simulink model "Ground_Control_SC"  (R2020b)
settings: Solver=VariableStepAuto  StartTime=0.0  StopTime=10.0  RelTol=1e-3
settings Model: Creator=macra  LastModifiedBy=macra

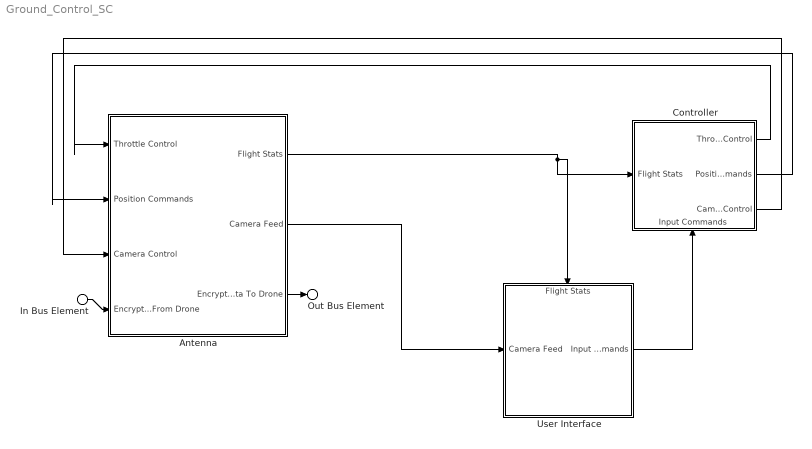
== system Ground_Control_SC ==
  In Bus Element : Inport  PortName=Encrypted Data From Drone
  Antenna : Subsystem
      settings: PortSchema="{\"entries\":[{\"content\":{\"headerSize\":26,\"margin\":15,\"minimumSpacing\":25,\"sides\":[{\"content\":{\"connectorIds\":[\"In1\",\"In2\",\"In3\",\"In4\"]},\"type\":\"ConnectorPlacement.EquallySpacedRectSide\",\"uuid\":\"8f51257f-f627-4f58-a4af-3e0fb88ba4bc\"},{\"content\":{\"connectorIds\":[\"Out1\",\"Out2\",\"Out3\"],\"side\":\"RIGHT\"},\"type\":\"ConnectorPlacement.EquallySpacedRectSide\",\"uuid\":\"f1fa1950-8e47-40b7-8d13-b3d0804be378\"},{\"content\":{\"connectorIds\":[],\"side\":\"TOP\"},\"type\":\"ConnectorPlacement.EquallySpacedRectSide\",\"uuid\":\"7a27bdc2-dc0c-4d7e-ba2c-0c757f448581\"},{\"content\":{\"connectorIds\":[],\"side\":\"HIDDEN\"},\"type\":\"ConnectorPlacement.EquallySpacedRectSide\",\"uuid\":\"bf1e85f7-7c79-4931-85e3-188682710bd5\"}]},\"type\":\"ConnectorPlacement.EquallySpacedConnector\",\"uuid\":\"5f8c8835-300e-4f03-b548-6a322d546785\"}],\"packageUris\":[\"http://schema.mathworks.com/mf0/Connector/R2020b\"],\"version\":\"1.0\"}"
  Controller : Subsystem
      settings: PortSchema="{\"entries\":[{\"content\":{\"headerSize\":26,\"margin\":15,\"minimumSpacing\":25,\"sides\":[{\"content\":{\"connectorIds\":[\"In1\"]},\"type\":\"ConnectorPlacement.EquallySpacedRectSide\",\"uuid\":\"8f51257f-f627-4f58-a4af-3e0fb88ba4bc\"},{\"content\":{\"connectorIds\":[\"Out1\",\"Out2\",\"Out3\"],\"side\":\"RIGHT\"},\"type\":\"ConnectorPlacement.EquallySpacedRectSide\",\"uuid\":\"f1fa1950-8e47-40b7-8d13-b3d0804be378\"},{\"content\":{\"connectorIds\":[],\"side\":\"TOP\"},\"type\":\"ConnectorPlacement.EquallySpacedRectSide\",\"uuid\":\"7a27bdc2-dc0c-4d7e-ba2c-0c757f448581\"},{\"content\":{\"connectorIds\":[\"In2\"],\"side\":\"BOTTOM\"},\"type\":\"ConnectorPlacement.EquallySpacedRectSide\",\"uuid\":\"100c20a7-19a0-4abc-9a19-4a6d998db79c\"},{\"content\":{\"connectorIds\":[],\"side\":\"HIDDEN\"},\"type\":\"ConnectorPlacement.EquallySpacedRectSide\",\"uuid\":\"bf1e85f7-7c79-4931-85e3-188682710bd5\"}]},\"type\":\"ConnectorPlacement.EquallySpacedConnector\",\"uuid\":\"5f8c8835-300e-4f03-b548-6a322d546785\"}],\"packageUris\":[\"http://schema.mathworks.com/mf0/Connector/R2020b\"],\"version\":\"1.0\"}"
  User Interface : Subsystem
      settings: PortSchema="{\"entries\":[{\"content\":{\"headerSize\":26,\"margin\":15,\"minimumSpacing\":25,\"sides\":[{\"content\":{\"connectorIds\":[\"In2\"]},\"type\":\"ConnectorPlacement.EquallySpacedRectSide\",\"uuid\":\"8f51257f-f627-4f58-a4af-3e0fb88ba4bc\"},{\"content\":{\"connectorIds\":[\"Out1\"],\"side\":\"RIGHT\"},\"type\":\"ConnectorPlacement.EquallySpacedRectSide\",\"uuid\":\"f1fa1950-8e47-40b7-8d13-b3d0804be378\"},{\"content\":{\"connectorIds\":[\"In1\"],\"side\":\"TOP\"},\"type\":\"ConnectorPlacement.EquallySpacedRectSide\",\"uuid\":\"7a27bdc2-dc0c-4d7e-ba2c-0c757f448581\"},{\"content\":{\"connectorIds\":[],\"side\":\"HIDDEN\"},\"type\":\"ConnectorPlacement.EquallySpacedRectSide\",\"uuid\":\"bf1e85f7-7c79-4931-85e3-188682710bd5\"}]},\"type\":\"ConnectorPlacement.EquallySpacedConnector\",\"uuid\":\"5f8c8835-300e-4f03-b548-6a322d546785\"}],\"packageUris\":[\"http://schema.mathworks.com/mf0/Connector/R2020b\"],\"version\":\"1.0\"}"
  Out Bus Element : Outport  PortName=Encrypted Data To Drone
  wires:
  Antenna/2(Camera Feed) -> User Interface/2(Camera Feed)
  User Interface/1(Input Commands) -> Controller/2(Input Commands)
  In Bus Element/1 -> Antenna/4(Encrypted Data From Drone)
  Antenna/3(Encrypted Data To Drone) -> Out Bus Element/1
  Antenna/1(Flight Stats) -> Controller/1(Flight Stats), User Interface/1(Flight Stats)
  Controller/1(Throttle Control) -> Antenna/1(Throttle Control)
  Controller/3(Camera Control) -> Antenna/3(Camera Control)
  Controller/2(Position Commands) -> Antenna/2(Position Commands)

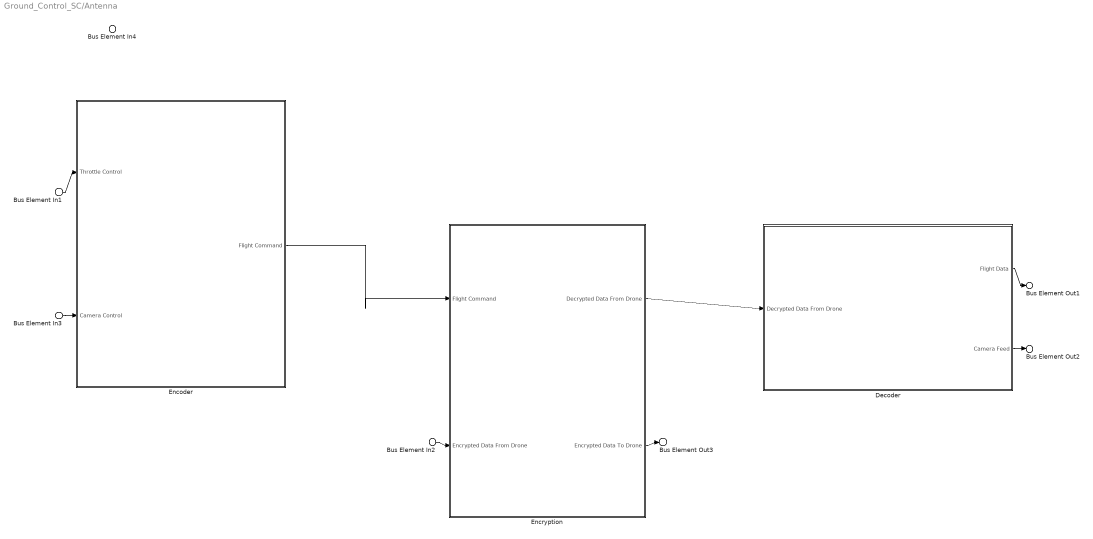
== system Ground_Control_SC/Antenna ==
  Bus Element In1 : Inport  PortName=Throttle Control
  Bus Element In4 : Inport  Port=2  PortName=Position Commands
  Bus Element In3 : Inport  Port=3  PortName=Camera Control
  Bus Element In2 : Inport  Port=4  PortName=Encrypted Data From Drone
  Decoder : Subsystem
      settings: PortSchema="{\"entries\":[{\"content\":{\"headerSize\":26,\"margin\":15,\"minimumSpacing\":25,\"sides\":[{\"content\":{\"connectorIds\":[\"In1\"]},\"type\":\"ConnectorPlacement.EquallySpacedRectSide\",\"uuid\":\"8f51257f-f627-4f58-a4af-3e0fb88ba4bc\"},{\"content\":{\"connectorIds\":[\"Out1\",\"Out2\"],\"side\":\"RIGHT\"},\"type\":\"ConnectorPlacement.EquallySpacedRectSide\",\"uuid\":\"f1fa1950-8e47-40b7-8d13-b3d0804be378\"},{\"content\":{\"connectorIds\":[],\"side\":\"TOP\"},\"type\":\"ConnectorPlacement.EquallySpacedRectSide\",\"uuid\":\"7a27bdc2-dc0c-4d7e-ba2c-0c757f448581\"},{\"content\":{\"connectorIds\":[],\"side\":\"HIDDEN\"},\"type\":\"ConnectorPlacement.EquallySpacedRectSide\",\"uuid\":\"bf1e85f7-7c79-4931-85e3-188682710bd5\"}]},\"type\":\"ConnectorPlacement.EquallySpacedConnector\",\"uuid\":\"5f8c8835-300e-4f03-b548-6a322d546785\"}],\"packageUris\":[\"http://schema.mathworks.com/mf0/Connector/R2020b\"],\"version\":\"1.0\"}"
  Encoder : Subsystem
      settings: PortSchema="{\"entries\":[{\"content\":{\"headerSize\":26,\"margin\":15,\"minimumSpacing\":25,\"sides\":[{\"content\":{\"connectorIds\":[\"In1\",\"In2\"]},\"type\":\"ConnectorPlacement.EquallySpacedRectSide\",\"uuid\":\"8f51257f-f627-4f58-a4af-3e0fb88ba4bc\"},{\"content\":{\"connectorIds\":[\"Out1\"],\"side\":\"RIGHT\"},\"type\":\"ConnectorPlacement.EquallySpacedRectSide\",\"uuid\":\"f1fa1950-8e47-40b7-8d13-b3d0804be378\"},{\"content\":{\"connectorIds\":[],\"side\":\"TOP\"},\"type\":\"ConnectorPlacement.EquallySpacedRectSide\",\"uuid\":\"7a27bdc2-dc0c-4d7e-ba2c-0c757f448581\"},{\"content\":{\"connectorIds\":[],\"side\":\"HIDDEN\"},\"type\":\"ConnectorPlacement.EquallySpacedRectSide\",\"uuid\":\"bf1e85f7-7c79-4931-85e3-188682710bd5\"}]},\"type\":\"ConnectorPlacement.EquallySpacedConnector\",\"uuid\":\"5f8c8835-300e-4f03-b548-6a322d546785\"}],\"packageUris\":[\"http://schema.mathworks.com/mf0/Connector/R2020b\"],\"version\":\"1.0\"}"
  Encryption : Subsystem
      settings: PortSchema="{\"entries\":[{\"content\":{\"headerSize\":26,\"margin\":15,\"minimumSpacing\":25,\"sides\":[{\"content\":{\"connectorIds\":[\"In1\",\"In2\"]},\"type\":\"ConnectorPlacement.EquallySpacedRectSide\",\"uuid\":\"8f51257f-f627-4f58-a4af-3e0fb88ba4bc\"},{\"content\":{\"connectorIds\":[\"Out1\",\"Out2\"],\"side\":\"RIGHT\"},\"type\":\"ConnectorPlacement.EquallySpacedRectSide\",\"uuid\":\"f1fa1950-8e47-40b7-8d13-b3d0804be378\"},{\"content\":{\"connectorIds\":[],\"side\":\"TOP\"},\"type\":\"ConnectorPlacement.EquallySpacedRectSide\",\"uuid\":\"7a27bdc2-dc0c-4d7e-ba2c-0c757f448581\"},{\"content\":{\"connectorIds\":[],\"side\":\"HIDDEN\"},\"type\":\"ConnectorPlacement.EquallySpacedRectSide\",\"uuid\":\"bf1e85f7-7c79-4931-85e3-188682710bd5\"}]},\"type\":\"ConnectorPlacement.EquallySpacedConnector\",\"uuid\":\"5f8c8835-300e-4f03-b548-6a322d546785\"}],\"packageUris\":[\"http://schema.mathworks.com/mf0/Connector/R2020b\"],\"version\":\"1.0\"}"
  Bus Element Out1 : Outport  PortName=Flight Stats
  Bus Element Out2 : Outport  Port=2  PortName=Camera Feed
  Bus Element Out3 : Outport  Port=3  PortName=Encrypted Data To Drone
  wires:
  Bus Element In2/1 -> Encryption/2(Encrypted Data From Drone)
  Encryption/2(Encrypted Data To Drone) -> Bus Element Out3/1
  Encryption/1(Decrypted Data From Drone) -> Decoder/1(Decrypted Data From Drone)
  Decoder/1(Flight Data) -> Bus Element Out1/1
  Decoder/2(Camera Feed) -> Bus Element Out2/1
  Encoder/1(Flight Command) -> Encryption/1(Flight Command)
  Bus Element In1/1 -> Encoder/1(Throttle Control)
  Bus Element In3/1 -> Encoder/2(Camera Control)

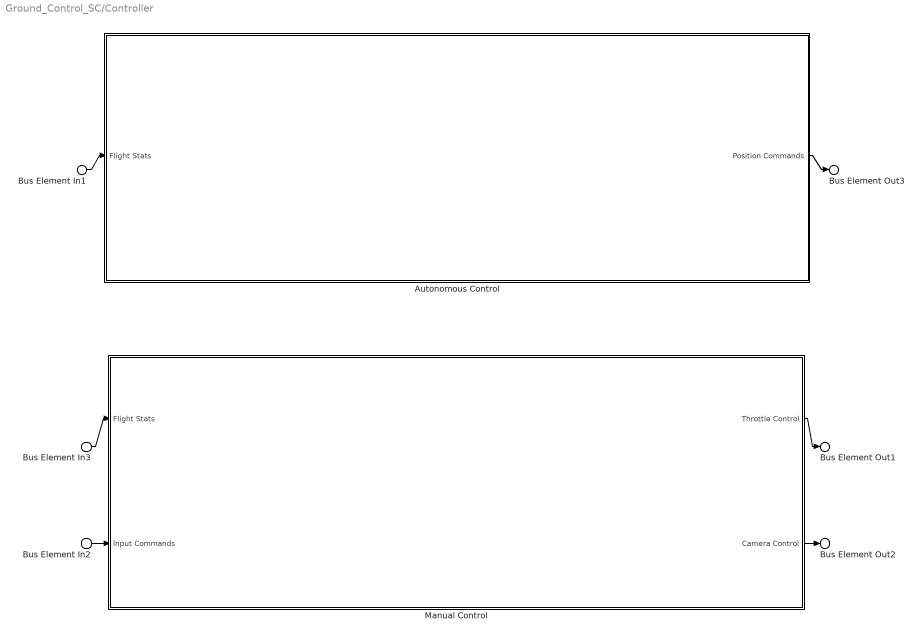
== system Ground_Control_SC/Controller ==
  Bus Element In1 : Inport  PortName=Flight Stats
  Bus Element In3 : Inport  PortName=Flight Stats
  Bus Element In2 : Inport  Port=2  PortName=Input Commands
  Autonomous Control : Subsystem
      settings: PortSchema="{\"entries\":[{\"content\":{\"headerSize\":26,\"margin\":15,\"minimumSpacing\":25,\"sides\":[{\"content\":{\"connectorIds\":[\"In1\"]},\"type\":\"ConnectorPlacement.EquallySpacedRectSide\",\"uuid\":\"8f51257f-f627-4f58-a4af-3e0fb88ba4bc\"},{\"content\":{\"connectorIds\":[\"Out1\"],\"side\":\"RIGHT\"},\"type\":\"ConnectorPlacement.EquallySpacedRectSide\",\"uuid\":\"f1fa1950-8e47-40b7-8d13-b3d0804be378\"},{\"content\":{\"connectorIds\":[],\"side\":\"TOP\"},\"type\":\"ConnectorPlacement.EquallySpacedRectSide\",\"uuid\":\"7a27bdc2-dc0c-4d7e-ba2c-0c757f448581\"},{\"content\":{\"connectorIds\":[],\"side\":\"HIDDEN\"},\"type\":\"ConnectorPlacement.EquallySpacedRectSide\",\"uuid\":\"bf1e85f7-7c79-4931-85e3-188682710bd5\"}]},\"type\":\"ConnectorPlacement.EquallySpacedConnector\",\"uuid\":\"5f8c8835-300e-4f03-b548-6a322d546785\"}],\"packageUris\":[\"http://schema.mathworks.com/mf0/Connector/R2020b\"],\"version\":\"1.0\"}"
  Manual Control : Subsystem
      settings: PortSchema="{\"entries\":[{\"content\":{\"headerSize\":26,\"margin\":15,\"minimumSpacing\":25,\"sides\":[{\"content\":{\"connectorIds\":[\"In1\",\"In2\"]},\"type\":\"ConnectorPlacement.EquallySpacedRectSide\",\"uuid\":\"8f51257f-f627-4f58-a4af-3e0fb88ba4bc\"},{\"content\":{\"connectorIds\":[\"Out1\",\"Out2\"],\"side\":\"RIGHT\"},\"type\":\"ConnectorPlacement.EquallySpacedRectSide\",\"uuid\":\"f1fa1950-8e47-40b7-8d13-b3d0804be378\"},{\"content\":{\"connectorIds\":[],\"side\":\"TOP\"},\"type\":\"ConnectorPlacement.EquallySpacedRectSide\",\"uuid\":\"7a27bdc2-dc0c-4d7e-ba2c-0c757f448581\"},{\"content\":{\"connectorIds\":[],\"side\":\"HIDDEN\"},\"type\":\"ConnectorPlacement.EquallySpacedRectSide\",\"uuid\":\"bf1e85f7-7c79-4931-85e3-188682710bd5\"}]},\"type\":\"ConnectorPlacement.EquallySpacedConnector\",\"uuid\":\"5f8c8835-300e-4f03-b548-6a322d546785\"}],\"packageUris\":[\"http://schema.mathworks.com/mf0/Connector/R2020b\"],\"version\":\"1.0\"}"
  Bus Element Out1 : Outport  PortName=Throttle Control
  Bus Element Out3 : Outport  Port=2  PortName=Position Commands
  Bus Element Out2 : Outport  Port=3  PortName=Camera Control
  wires:
  Bus Element In1/1 -> Autonomous Control/1(Flight Stats)
  Bus Element In3/1 -> Manual Control/1(Flight Stats)
  Bus Element In2/1 -> Manual Control/2(Input Commands)
  Manual Control/2(Camera Control) -> Bus Element Out2/1
  Autonomous Control/1(Position Commands) -> Bus Element Out3/1
  Manual Control/1(Throttle Control) -> Bus Element Out1/1

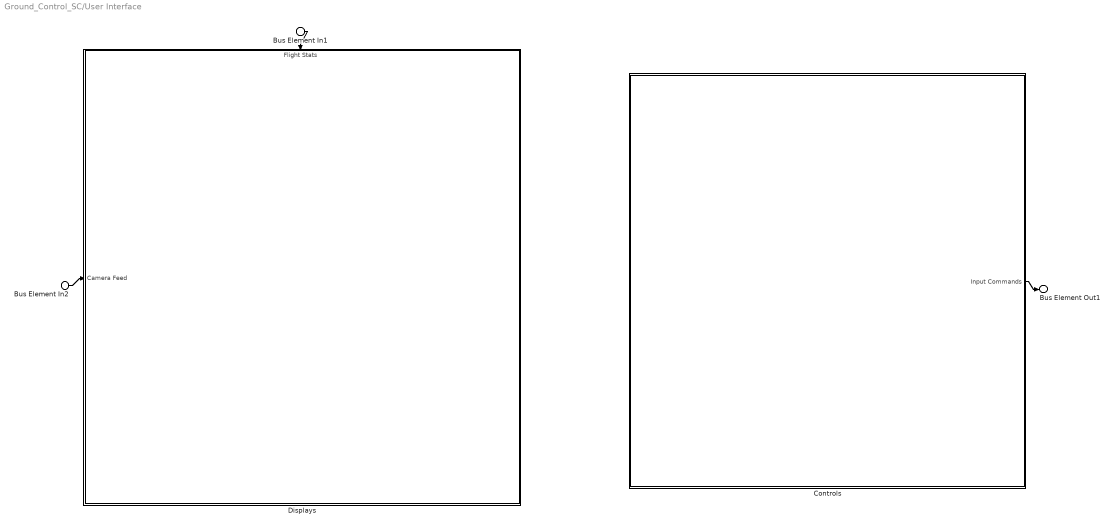
== system Ground_Control_SC/User Interface ==
  Bus Element In1 : Inport  PortName=Flight Stats
  Bus Element In2 : Inport  Port=2  PortName=Camera Feed
  Controls : Subsystem
      settings: PortSchema="{\"entries\":[{\"content\":{\"headerSize\":26,\"margin\":15,\"minimumSpacing\":25,\"sides\":[{\"content\":{\"connectorIds\":[]},\"type\":\"ConnectorPlacement.EquallySpacedRectSide\",\"uuid\":\"8f51257f-f627-4f58-a4af-3e0fb88ba4bc\"},{\"content\":{\"connectorIds\":[\"Out1\"],\"side\":\"RIGHT\"},\"type\":\"ConnectorPlacement.EquallySpacedRectSide\",\"uuid\":\"f1fa1950-8e47-40b7-8d13-b3d0804be378\"},{\"content\":{\"connectorIds\":[],\"side\":\"TOP\"},\"type\":\"ConnectorPlacement.EquallySpacedRectSide\",\"uuid\":\"7a27bdc2-dc0c-4d7e-ba2c-0c757f448581\"},{\"content\":{\"connectorIds\":[],\"side\":\"HIDDEN\"},\"type\":\"ConnectorPlacement.EquallySpacedRectSide\",\"uuid\":\"bf1e85f7-7c79-4931-85e3-188682710bd5\"}]},\"type\":\"ConnectorPlacement.EquallySpacedConnector\",\"uuid\":\"5f8c8835-300e-4f03-b548-6a322d546785\"}],\"packageUris\":[\"http://schema.mathworks.com/mf0/Connector/R2020b\"],\"version\":\"1.0\"}"
  Displays : Subsystem
      settings: PortSchema="{\"entries\":[{\"content\":{\"headerSize\":26,\"margin\":15,\"minimumSpacing\":25,\"sides\":[{\"content\":{\"connectorIds\":[\"In1\"]},\"type\":\"ConnectorPlacement.EquallySpacedRectSide\",\"uuid\":\"8f51257f-f627-4f58-a4af-3e0fb88ba4bc\"},{\"content\":{\"connectorIds\":[],\"side\":\"RIGHT\"},\"type\":\"ConnectorPlacement.EquallySpacedRectSide\",\"uuid\":\"f1fa1950-8e47-40b7-8d13-b3d0804be378\"},{\"content\":{\"connectorIds\":[\"In2\"],\"side\":\"TOP\"},\"type\":\"ConnectorPlacement.EquallySpacedRectSide\",\"uuid\":\"7a27bdc2-dc0c-4d7e-ba2c-0c757f448581\"},{\"content\":{\"connectorIds\":[],\"side\":\"HIDDEN\"},\"type\":\"ConnectorPlacement.EquallySpacedRectSide\",\"uuid\":\"bf1e85f7-7c79-4931-85e3-188682710bd5\"}]},\"type\":\"ConnectorPlacement.EquallySpacedConnector\",\"uuid\":\"5f8c8835-300e-4f03-b548-6a322d546785\"}],\"packageUris\":[\"http://schema.mathworks.com/mf0/Connector/R2020b\"],\"version\":\"1.0\"}"
  Bus Element Out1 : Outport  PortName=Input Commands
  wires:
  Bus Element In1/1 -> Displays/2(Flight Stats)
  Bus Element In2/1 -> Displays/1(Camera Feed)
  Controls/1(Input Commands) -> Bus Element Out1/1

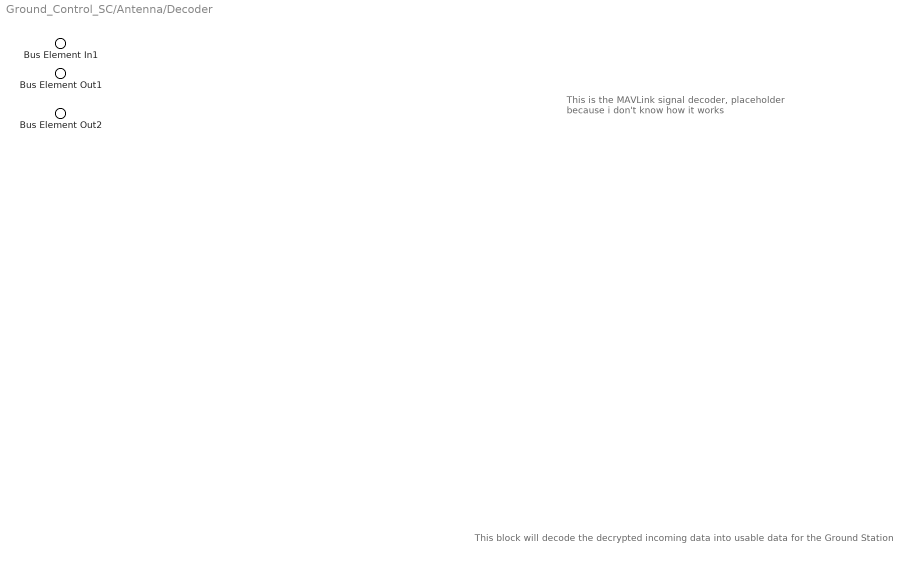
== system Ground_Control_SC/Antenna/Decoder ==
  note: This is the MAVLink signal decoder, placeholder
      | because i don't know how it works
  note: This block will decode the decrypted incoming data into usable data for the Ground Station
  Bus Element In1 : Inport  PortName=Decrypted Data From Drone
  Bus Element Out1 : Outport  PortName=Flight Data
  Bus Element Out2 : Outport  Port=2  PortName=Camera Feed

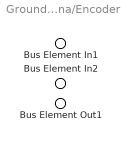
== system Ground_Control_SC/Antenna/Encoder ==
  Bus Element In1 : Inport  PortName=Throttle Control
  Bus Element In2 : Inport  Port=2  PortName=Camera Control
  Bus Element Out1 : Outport  PortName=Flight Command

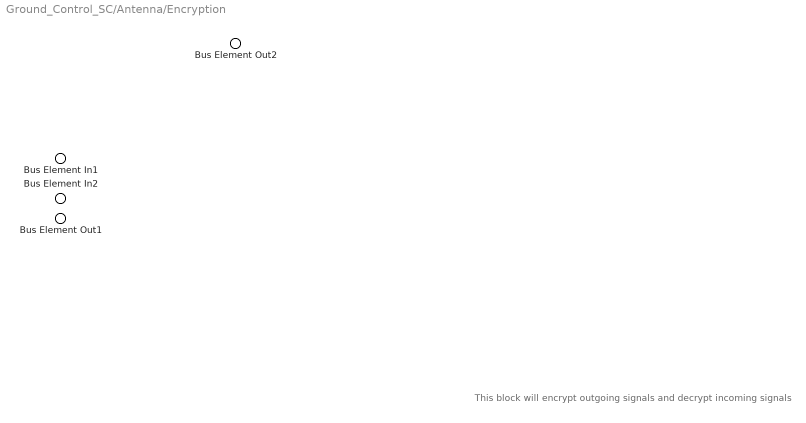
== system Ground_Control_SC/Antenna/Encryption ==
  note: This block will encrypt outgoing signals and decrypt incoming signals
  Bus Element In1 : Inport  PortName=Flight Command
  Bus Element In2 : Inport  Port=2  PortName=Encrypted Data From Drone
  Bus Element Out2 : Outport  PortName=Decrypted Data From Drone
  Bus Element Out1 : Outport  Port=2  PortName=Encrypted Data To Drone

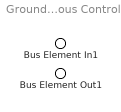
== system Ground_Control_SC/Controller/Autonomous Control ==
  Bus Element In1 : Inport  PortName=Flight Stats
  Bus Element Out1 : Outport  PortName=Position Commands

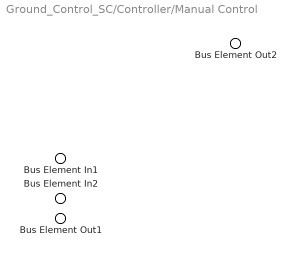
== system Ground_Control_SC/Controller/Manual Control ==
  Bus Element In1 : Inport  PortName=Flight Stats
  Bus Element In2 : Inport  Port=2  PortName=Input Commands
  Bus Element Out2 : Outport  PortName=Throttle Control
  Bus Element Out1 : Outport  Port=2  PortName=Camera Control

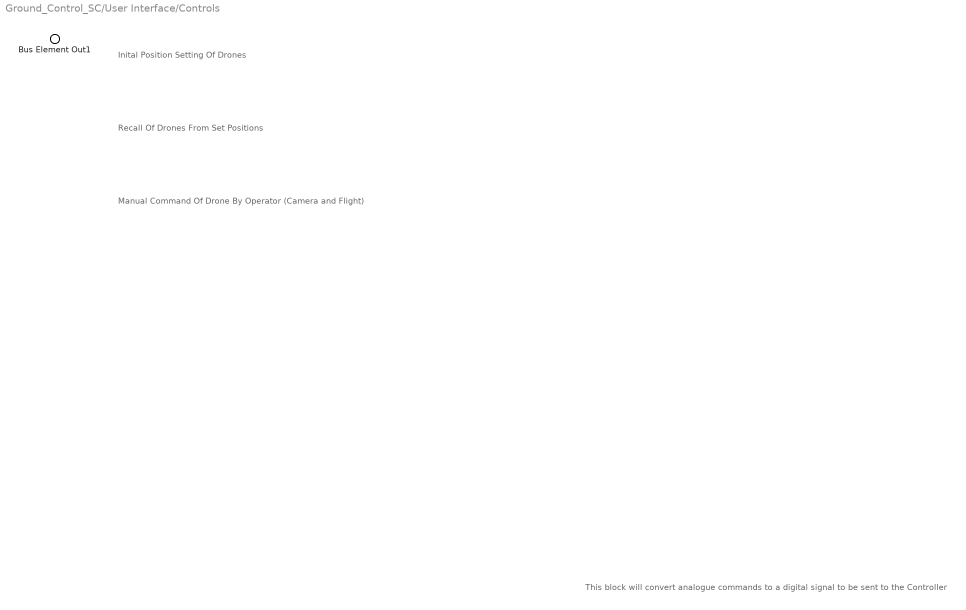
== system Ground_Control_SC/User Interface/Controls ==
  note: This block will convert analogue commands to a digital signal to be sent to the Controller
  note: Inital Position Setting Of Drones
  note: Recall Of Drones From Set Positions
  note: Manual Command Of Drone By Operator (Camera and Flight)
  Bus Element Out1 : Outport  PortName=Input Commands

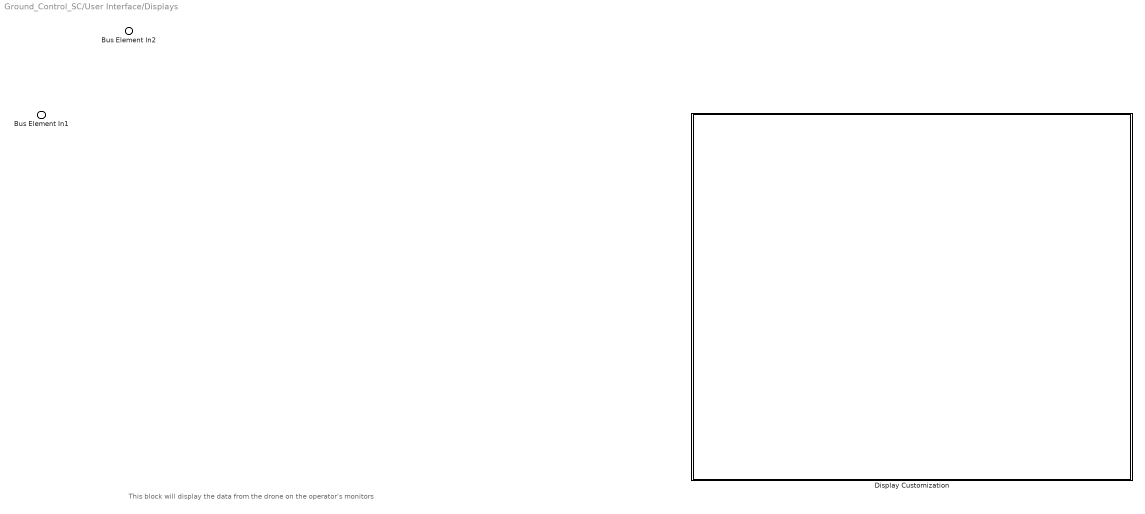
== system Ground_Control_SC/User Interface/Displays ==
  note: This block will display the data from the drone on the operator's monitors
  Bus Element In2 : Inport  PortName=Camera Feed
  Bus Element In1 : Inport  Port=2  PortName=Flight Stats
  Display Customization : Subsystem
      settings: PortSchema="{\"entries\":[{\"content\":{\"headerSize\":26,\"margin\":15,\"minimumSpacing\":25,\"sides\":[{\"content\":{\"connectorIds\":[]},\"type\":\"ConnectorPlacement.EquallySpacedRectSide\",\"uuid\":\"8f51257f-f627-4f58-a4af-3e0fb88ba4bc\"},{\"content\":{\"connectorIds\":[],\"side\":\"RIGHT\"},\"type\":\"ConnectorPlacement.EquallySpacedRectSide\",\"uuid\":\"f1fa1950-8e47-40b7-8d13-b3d0804be378\"},{\"content\":{\"connectorIds\":[],\"side\":\"TOP\"},\"type\":\"ConnectorPlacement.EquallySpacedRectSide\",\"uuid\":\"7a27bdc2-dc0c-4d7e-ba2c-0c757f448581\"},{\"content\":{\"connectorIds\":[],\"side\":\"HIDDEN\"},\"type\":\"ConnectorPlacement.EquallySpacedRectSide\",\"uuid\":\"bf1e85f7-7c79-4931-85e3-188682710bd5\"}]},\"type\":\"ConnectorPlacement.EquallySpacedConnector\",\"uuid\":\"5f8c8835-300e-4f03-b548-6a322d546785\"}],\"packageUris\":[\"http://schema.mathworks.com/mf0/Connector/R2020b\"],\"version\":\"1.0\"}"

== system Ground_Control_SC/User Interface/Displays/Display Customization ==
  note: This block will allow the display configuration to be customized
